simulink subsystem "subsystem_event_top_trig_simplified"  (R2022a)
settings: Solver=VariableStepAuto  StartTime=0.0  StopTime=10.0  RelTol=1e-3
undefined symbols (not defined in the file): rel_diff, timescale
libraries: neuromorphic_blocks x6
settings Model: Creator=chris  LastModifiedBy=chris

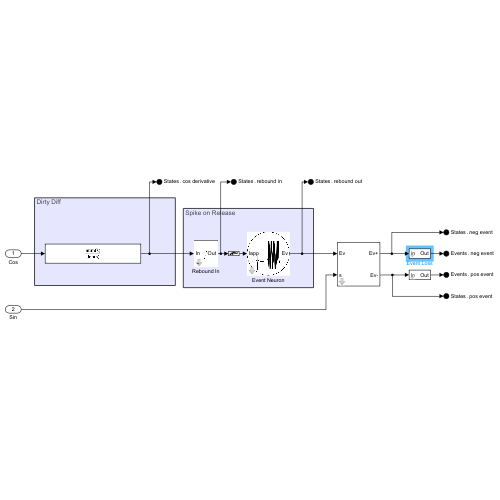
[thumbnail: Simulink's stored preview of the top-level diagram]
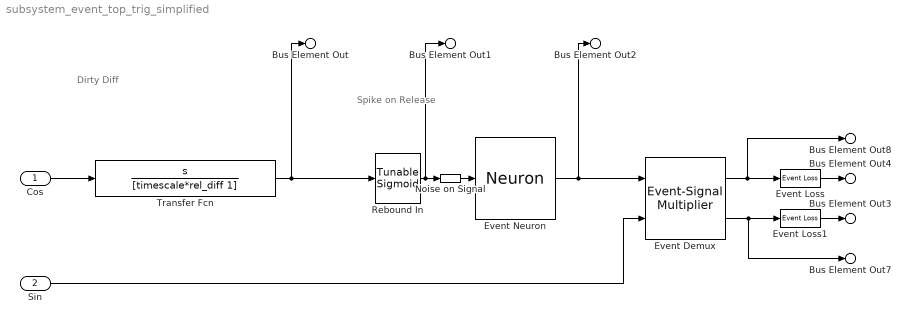
== system subsystem_event_top_trig_simplified ==
  note: Dirty Diff
  note: Spike on Release
  Cos : Inport
  Sin : Inport  Port=2
  Event Demux : neuromorphic_blocks/Auxiliary Blocks/Event-Signal Multiplier  symmetric_box=off  dsyn_signal_pos=10  dsyn_signal_neg=10  dsyn_signal_neg_save=10  gain_signal_pos=100  gain_signal_neg=100  gain_signal_neg_save=100  input=Events  gsyn_pos=20  gsyn_neg=20  gsyn_neg_save=20  dsyn_event_pos=0  dsyn_event_neg=0  dsyn_event_neg_save=0  gain_event_pos=20  gain_event_neg=20  gain_event_neg_save=20
      settings: SourceProductName=NeurCont Toolbox
  Event Loss : neuromorphic_blocks/Events Transmission Blocks/Event Loss  loss_prob=prob_event_loss  seed=-1  seed_mem=randi([0, 100000])
      settings: SourceProductName=Neuromorphic Toolbox
  Event Loss1 : neuromorphic_blocks/Events Transmission Blocks/Event Loss  loss_prob=prob_event_loss  seed=-1  seed_mem=randi([0, 100000])
      settings: SourceProductName=Neuromorphic Toolbox
  Event Neuron : neuromorphic_blocks/Neural Blocks/Neuron  gfm_source=Internal  gfm=3  gsp_source=Internal  gsp=10  gsm_source=Internal  gsm=0  gup_source=Internal  gup=0  gum_source=Internal  gum=0  dfm=0  dsp=0.5  dsm=-0.5  dup=-0.5  dum=-1  mfm=1  msp=1  msm=1  mup=1  mum=1  timescale=timescale  rel_membrane=0.1  rel_fast=0.1  rel_slow=4  rel_ultraslow=200  Iapp_base=0.0  V0=-1.2  tresh=0.0  output=Events
      settings: SourceProductName=Neuromorphic Toolbox
  Noise on Signal : neuromorphic_blocks/Auxiliary Blocks/Noise on Signal  noise_pwr=noisePwr  timescale=timescale  rel_timescale=rel_noise  seed=-1  seed_mem=randi([0, 100000])
      settings: SourceProductName=NeurCont Toolbox
  Rebound In : neuromorphic_blocks/Tunable Sigmoid  nonlinearity_type=Sigmoid  gain_source=Internal  gain=-1.5  bias=5  slope=-100
      settings: SourceProductName=Neuromorphic Toolbox
  Transfer Fcn : TransferFcn  Numerator=[1 0]  Denominator=[timescale*rel_diff 1]
  Bus Element Out3 : Outport  PortName=Events  Element=pos event
  Bus Element Out4 : Outport  PortName=Events  Element=neg event
  Bus Element Out : Outport  Port=2  PortName=States  Element=cos derivative
  Bus Element Out1 : Outport  Port=2  PortName=States  Element=rebound in
  Bus Element Out2 : Outport  Port=2  PortName=States  Element=rebound out
  Bus Element Out7 : Outport  Port=2  PortName=States  Element=pos event
  Bus Element Out8 : Outport  Port=2  PortName=States  Element=neg event
  wires:
  Rebound In/1 -> Noise on Signal/1, Bus Element Out1/1
  Cos/1 -> Transfer Fcn/1
  Transfer Fcn/1 -> Rebound In/1, Bus Element Out/1
  Event Neuron/1 -> Bus Element Out2/1, Event Demux/1
  Event Demux/2 -> Bus Element Out7/1, Event Loss1/1
  Event Demux/1 -> Bus Element Out8/1, Event Loss/1
  Event Loss1/1 -> Bus Element Out3/1
  Event Loss/1 -> Bus Element Out4/1
  Noise on Signal/1 -> Event Neuron/1
  Sin/1 -> Event Demux/2
